simulink model "suivi_points"  (R2021b)
settings: Solver=VariableStepAuto  StartTime=0.0  StopTime=100.0  RelTol=1e-3
values from neighbouring files (symbols this model uses):
  a1mot = -lambdamot    [fichierconfig.m]
  alphainit = 3.14/2    (= 1.57)    [fichierconfig.m]
  b1mot = G*(1-lambdamot)    [fichierconfig.m]
  L = 0.0865    [fichierconfig.m]
  paramIangle = (r1angle+r0angle)/Te    (= 1.25)    [fichierconfig.m]
  paramImoteur = (r1+r0)/Te    (= 2.95980583674)    [fichierconfig.m]
  paramPangle = r0angle    (= 0.1625)    [fichierconfig.m]
  paramPmoteur = r0    (= 0.384774758776)    [fichierconfig.m]
  Pxcible = +0.5    (= 0.5)    [fichierconfig.m]
  Pxinit = 0    [fichierconfig.m]
  Pycible = -0.5    [fichierconfig.m]
  Pyinit = 0    [fichierconfig.m]
  r = 0.030    (= 0.03)    [fichierconfig.m]
  Te = 0.040    (= 0.04)    [fichierconfig.m]
undefined symbols (not defined in the file or in its folder): DiscIntNeverNeededParam
libraries: slpidlib x3, simulink x1
settings Model: Creator=mlouaze  LastModifiedBy=mlouaze

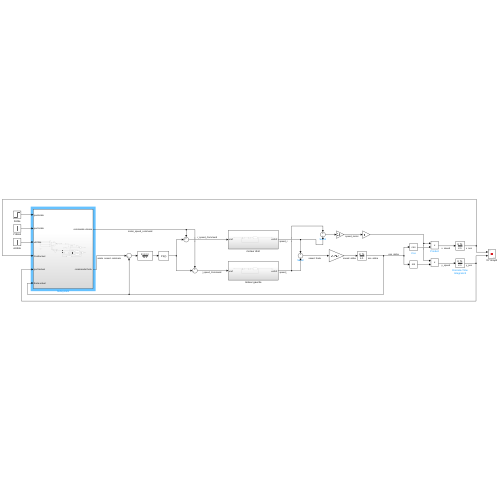
[thumbnail: Simulink's stored preview of the top-level diagram]
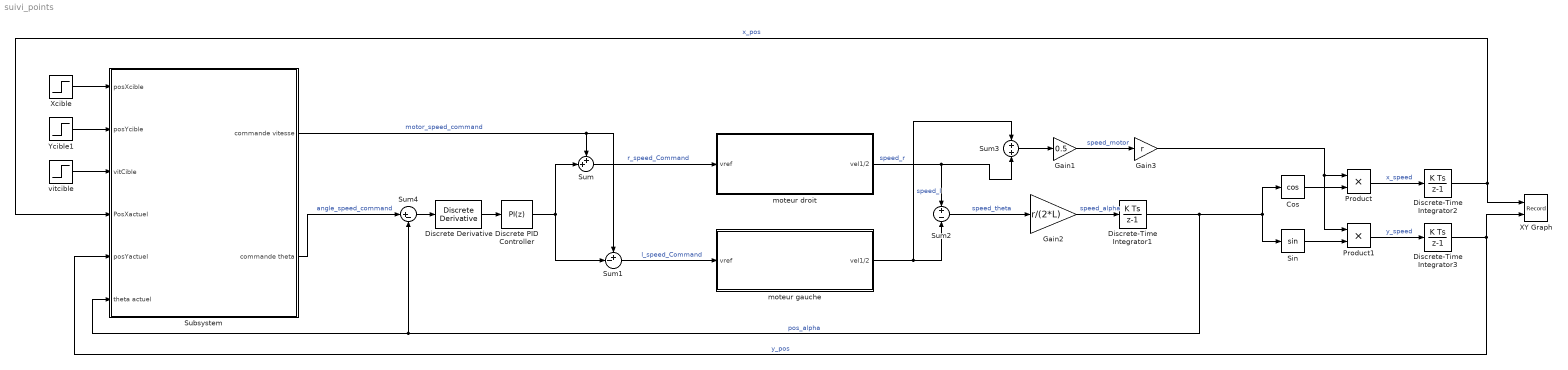
== system suivi_points ==
  Cos : Trigonometry  Operator=cos
  Discrete Derivative : simulink/Discrete/Discrete Derivative  gainval=1.0  ICPrevScaledInput=0.0  OutMin=[]  OutMax=[]  OutDataType=fixdt(1, 16)  OutScaling=2^-10  DoSatur=off
  Discrete PID Controller : slpidlib/PID Controller  Controller=PI  Form=Parallel  TimeDomain=Discrete-time  UseExternalTs=off  SampleTime=-1  IntegratorMethod=Forward Euler  FilterMethod=Forward Euler  ControllerParametersSource=internal  P=paramPangle  I=paramIangle  D=0  UseFilter=on  N=100  TunerSelectOption=Transfer Function Based (PID Tuner App)  InitialConditionSource=internal  InitialConditionForIntegrator=0  InitialConditionForFilter=0  DifferentiatorICPrevScaledInput=0  ExternalReset=none  TrackingMode=off  Kt=1  LimitOutput=off  SatLimitsSource=internal  UpperSaturationLimit=inf  LowerSaturationLimit=-inf  LinearizeAsGain=off  AntiWindupMode=none  Kb=1  POutMin=[]  POutMax=[]  IOutMin=[]  IOutMax=[]  DOutMin=[]  DOutMax=[]  NOutMin=[]  NOutMax=[]  SumOutMin=[]  SumOutMax=[]  SaturationOutMin=[]  SaturationOutMax=[]  PParamMin=[]  PParamMax=[]  IParamMin=[]  IParamMax=[]  DParamMin=[]  DParamMax=[]  NParamMin=[]  NParamMax=[]  KbParamMin=[]  KbParamMax=[]  KtParamMin=[]  KtParamMax=[]  KbOutMin=[]  KbOutMax=[]  KtOutMin=[]  KtOutMax=[]  IntegratorOutMin=[]  IntegratorOutMax=[]  FilterOutMin=[]  FilterOutMax=[]  SumI1OutMin=[]  SumI1OutMax=[]  SumI2OutMin=[]  SumI2OutMax=[]  SumI3OutMin=[]  SumI3OutMax=[]  SumI4OutMin=[]  SumI4OutMax=[]  SumDOutMin=[]  SumDOutMax=[]  DifferentiatorOutMin=[]  DifferentiatorOutMax=[]  FilterDiffOutCoefMin=[]  FilterDiffOutCoefMax=[]  ReciprocalOutMin=[]  ReciprocalOutMax=[]  SumDenOutMin=[]  SumDenOutMax=[]  SumNumOutMin=[]  SumNumOutMax=[]  DivideOutMin=[]  DivideOutMax=[]  UdiffTsProdOutMin=[]  UdiffTsProdOutMax=[]  NTsProdOutMin=[]  NTsProdOutMax=[]  UintegralTsProdOutMin=[]  UintegralTsProdOutMax=[]  UngainTsProdOutMin=[]  UngainTsProdOutMax=[]  IntegratorContinuousStateAttributes=''  IntegratorStateMustResolveToSignalObject=off  IntegratorRTWStateStorageClass=Auto  FilterContinuousStateAttributes=''  FilterStateMustResolveToSignalObject=off  FilterRTWStateStorageClass=Auto  ParallelPVariant=InternalParameters  IdealPVariant=Disabled  IVariant=InternalParameters  DVariant=Disabled  IntegratorVariant=Discrete  SatVariant=Disabled  AWVariant=Passthrough  PCopyVariant=Disabled  TRVariant=Disabled  FdbkBlocksVariant=Forward  IdealPFdbkVariant=Disabled  SatFdbkVariant=Disabled  DerivativeFilterVariant=Disabled  NVariant=Disabled  NCopyVariant=Disabled_SignalSpec  FilterICVariant=Disabled  IntegratorICVariant=InternalICs  ExternalResetVariant=Disabled  TRSumVariant=Passthrough  SumFdbkVariant=Disabled  SumVariant=Sum_PI  TsampFilterVariant=InternalTs  TsampNgainVariant=Passthrough  TsampIntegralVariant=Passthrough  ExternalSaturationOutDataTypeStr=Inherit: Same as second input
  Discrete-Time Integrator1 : DiscreteIntegrator  InitialCondition=alphainit  SampleTime=-1  ICPrevOutput=DiscIntNeverNeededParam  ICPrevScaledInput=DiscIntNeverNeededParam
  Discrete-Time Integrator2 : DiscreteIntegrator  InitialCondition=Pxinit  SampleTime=-1  ICPrevOutput=DiscIntNeverNeededParam  ICPrevScaledInput=DiscIntNeverNeededParam
  Discrete-Time Integrator3 : DiscreteIntegrator  InitialCondition=Pyinit  SampleTime=-1  ICPrevOutput=DiscIntNeverNeededParam  ICPrevScaledInput=DiscIntNeverNeededParam
  Gain1 : Gain  Gain=0.5
  Gain2 : Gain  Gain=r/(2*L)
  Gain3 : Gain  Gain=r
  Product : Product
  Product1 : Product
  Sin : Trigonometry
  Subsystem : Subsystem
  Sum : Sum  Inputs=++|
  Sum1 : Sum  Inputs=+-|
  Sum2 : Sum  Inputs=+|-
  Sum3 : Sum  Inputs=+|+
  Sum4 : Sum  Inputs=|+-
  XY Graph : Record  FileSettingsInternal="{\"entries\":[{\"content\":{\"excelSettings\":{\"content\":{},\"type\":\"Streamout.ExcelSettings\"}},\"type\":\"Streamout.FileSettingStorage\",\"uuid\":\"98866556-d0f7-486d-9cf8-d99074070bc6\"}],\"packageUris\":[\"http://schema.mathworks.com/mf0/streamout_blocks/R2020a\"],\"version\":\"1.0\"}"  Layout=[1 1]  SignalsInternal="{\"entries\":[{\"content\":{\"signals\":[{\"content\":{\"blockPath\":[\"suivi_points/XY Graph\"],\"channel\":[],\"dimensions\":[1],\"domain\":\"suivi_points/XY Graph\",\"lineColor\":\"#a2142f\",\"plots\":[1],\"port\":1,\"sid\":[],\"signalID\":195,\"signalName\":\"x_pos\"},\"type\":\"RecordBlkView.Signal\",\"uuid\":\"87e10cd6-bcd0-46b1-8b3f-b12dfa0b8648\"},{\"content\":{\"blockPath\":[\"suivi_points/XY Graph\"],\"channel\":[],\"dimensions\":[1],\"domain\":\"suivi_points/XY Graph\",\"lineColor\":\"#139fff\",\"plots\":[1],\"port\":2,\"sid\":[],\"signalID\":198,\"signalName\":\"y_pos\"},\"type\":\"RecordBlkView.Signal\",\"uuid\":\"d70f9b69-a242-43ad-b3a3-1026d45bf527\"}]},\"type\":\"RecordBlkView.InputSignals\",\"uuid\":\"c4c30806-3f6a-4c2f-8db3-67a8f3bce1fd\"}],\"packageUris\":[\"http://schema.mathworks.com/mf0/streamout_blocks/R2020a\"],\"version\":\"1.0\"}"  VisualizationBindings="{\"xyplotplugin\":{\"info\":[{\"series\":[{\"bindingParametersList\":[{\"parameter\":\"X-Axis\",\"signalID\":195,\"signalName\":\"x_pos\"},{\"parameter\":\"Y-Axis\",\"signalID\":198,\"signalName\":\"y_pos\"}],\"seriesID\":64413}],\"subplotID\":1}]}}"  CompatibilityTag=XY  st=-1
  Xcible : Step  Time=0  After=Pxcible  SampleTime=Te
  Ycible1 : Step  Time=0  After=Pycible  SampleTime=Te
  moteur droit : Subsystem
  moteur gauche : Subsystem
  vitcible : Step  Time=0  SampleTime=Te
  wires:
  Sum3/1 -> Gain1/1
  Xcible/1 -> Subsystem/1(posXcible)
  Cos/1 -> Product/2
  Ycible1/1 -> Subsystem/2(posYcible)
  Sum2/1 -> Gain2/1  "speed_theta"
  Product/1 -> Discrete-Time Integrator2/1  "x_speed"
  Subsystem/1(commande vitesse) -> Sum1/1, Sum/1  "motor_speed_command"
  Discrete PID Controller/1 -> Sum/2, Sum1/2
  Subsystem/2("commande theta ") -> Sum4/1  "angle_speed_command"
  moteur droit/1(vel1/2) -> Sum3/2, Sum2/1  "speed_r"
  moteur gauche/1(vel1/2) -> Sum2/2, Sum3/1  "speed_l"
  Discrete-Time Integrator1/1 -> Cos/1, Sin/1, Subsystem/6(theta actuel), Sum4/2  "pos_alpha"
  Gain2/1 -> Discrete-Time Integrator1/1  "speed_alpha"
  Discrete-Time Integrator3/1 -> XY Graph/2, Subsystem/5(posYactuel)  "y_pos"
  Sum1/1 -> moteur gauche/1(vref)  "l_speed_Command"
  Sin/1 -> Product1/2
  Sum/1 -> moteur droit/1(vref)  "r_speed_Command"
  Gain3/1 -> Product1/1, Product/1
  Product1/1 -> Discrete-Time Integrator3/1  "y_speed"
  Discrete-Time Integrator2/1 -> XY Graph/1, Subsystem/4(PosXactuel)  "x_pos"
  Gain1/1 -> Gain3/1  "speed_motor"
  vitcible/1 -> Subsystem/3(vitCible)
  Discrete Derivative/1 -> Discrete PID Controller/1
  Sum4/1 -> Discrete Derivative/1

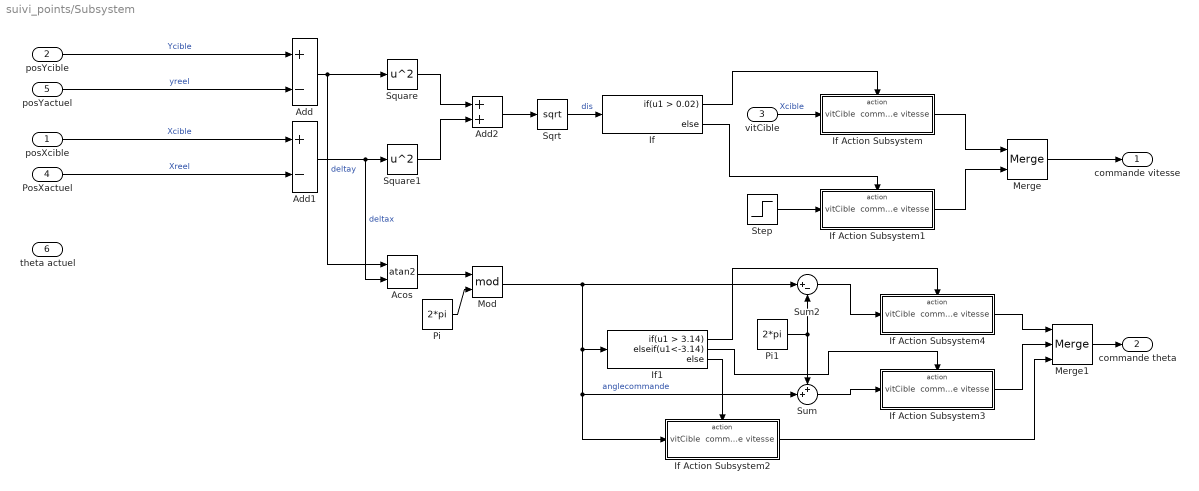
== system suivi_points/Subsystem ==
  posXcible : Inport
  posYcible : Inport  Port=2
  vitCible : Inport  Port=3
  PosXactuel : Inport  Port=4
  posYactuel : Inport  Port=5
  theta actuel : Inport  Port=6
  Acos : Trigonometry  Operator=atan2
  Add : Sum  Inputs=+-
  Add1 : Sum  Inputs=+-
  Add2 : Sum
  If : If  IfExpression=u1 > 0.02
  If Action Subsystem : Subsystem  TreatAsAtomicUnit=on
  If Action Subsystem1 : Subsystem  TreatAsAtomicUnit=on
  If Action Subsystem2 : Subsystem  TreatAsAtomicUnit=on
  If Action Subsystem3 : Subsystem  TreatAsAtomicUnit=on
  If Action Subsystem4 : Subsystem  TreatAsAtomicUnit=on
  If1 : If  IfExpression=u1 > 3.14  ElseIfExpressions=u1<-3.14
  Merge : Merge
  Merge1 : Merge  Inputs=3
  Mod : Math  Operator=mod  SaturateOnIntegerOverflow=on
  Pi : Constant  Value=2*pi  OutDataTypeStr=Inherit: Inherit via back propagation  SampleTime=-1
  Pi1 : Constant  Value=2*pi  OutDataTypeStr=Inherit: Inherit via back propagation
  Sqrt : Sqrt  SaturateOnIntegerOverflow=on
  Square : Math  Operator=square  SaturateOnIntegerOverflow=on
  Square1 : Math  Operator=square  SaturateOnIntegerOverflow=on
  Step : Step  Time=0  After=0  SampleTime=0
  Sum : Sum  Inputs=++|
  Sum2 : Sum  Inputs=|+-
  commande vitesse : Outport
  "commande theta " : Outport  Port=2
  wires:
  posYcible/1 -> Add/1  "Ycible"
  posYactuel/1 -> Add/2  "yreel"
  posXcible/1 -> Add1/1  "Xcible"
  PosXactuel/1 -> Add1/2  "Xreel"
  Add/1 -> Acos/1, Square/1  "deltay"
  Add1/1 -> Square1/1, Acos/2  "deltax"
  Square1/1 -> Add2/2
  Square/1 -> Add2/1
  Add2/1 -> Sqrt/1
  Sqrt/1 -> If/1  "dis"
  Mod/1 -> If Action Subsystem2/1(vitCible), Sum/2, If1/1, Sum2/1  "anglecommande"
  Merge1/1 -> "commande theta "/1
  vitCible/1 -> If Action Subsystem/1(vitCible)  "Xcible"
  If/1 -> If Action Subsystem/Action
  If/2 -> If Action Subsystem1/Action
  Step/1 -> If Action Subsystem1/1(vitCible)
  Merge/1 -> commande vitesse/1
  If Action Subsystem1/1(commande vitesse) -> Merge/2
  Acos/1 -> Mod/1
  Pi/1 -> Mod/2
  If1/3 -> If Action Subsystem2/Action
  If Action Subsystem2/1(commande vitesse) -> Merge1/3
  If1/2 -> If Action Subsystem3/Action
  If Action Subsystem3/1(commande vitesse) -> Merge1/2
  Sum/1 -> If Action Subsystem3/1(vitCible)
  If1/1 -> If Action Subsystem4/Action
  If Action Subsystem4/1(commande vitesse) -> Merge1/1
  Sum2/1 -> If Action Subsystem4/1(vitCible)
  Pi1/1 -> Sum/1, Sum2/2
  If Action Subsystem/1(commande vitesse) -> Merge/1

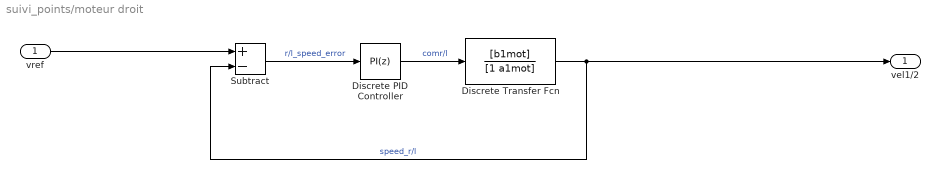
== system suivi_points/moteur droit ==
  vref : Inport
  Discrete Transfer Fcn : DiscreteTransferFcn  Numerator=[b1mot]  Denominator=[1 a1mot]
  Discrete PID Controller : slpidlib/PID Controller  Controller=PI  Form=Parallel  TimeDomain=Discrete-time  UseExternalTs=off  SampleTime=-1  IntegratorMethod=Forward Euler  FilterMethod=Forward Euler  ControllerParametersSource=internal  P=paramPmoteur  I=paramImoteur  D=0  UseFilter=on  N=100  TunerSelectOption=Transfer Function Based (PID Tuner App)  InitialConditionSource=internal  InitialConditionForIntegrator=0  InitialConditionForFilter=0  DifferentiatorICPrevScaledInput=0  ExternalReset=none  TrackingMode=off  Kt=1  LimitOutput=off  SatLimitsSource=internal  UpperSaturationLimit=inf  LowerSaturationLimit=-inf  LinearizeAsGain=off  AntiWindupMode=none  Kb=1  POutMin=[]  POutMax=[]  IOutMin=[]  IOutMax=[]  DOutMin=[]  DOutMax=[]  NOutMin=[]  NOutMax=[]  SumOutMin=[]  SumOutMax=[]  SaturationOutMin=[]  SaturationOutMax=[]  PParamMin=[]  PParamMax=[]  IParamMin=[]  IParamMax=[]  DParamMin=[]  DParamMax=[]  NParamMin=[]  NParamMax=[]  KbParamMin=[]  KbParamMax=[]  KtParamMin=[]  KtParamMax=[]  KbOutMin=[]  KbOutMax=[]  KtOutMin=[]  KtOutMax=[]  IntegratorOutMin=[]  IntegratorOutMax=[]  FilterOutMin=[]  FilterOutMax=[]  SumI1OutMin=[]  SumI1OutMax=[]  SumI2OutMin=[]  SumI2OutMax=[]  SumI3OutMin=[]  SumI3OutMax=[]  SumI4OutMin=[]  SumI4OutMax=[]  SumDOutMin=[]  SumDOutMax=[]  DifferentiatorOutMin=[]  DifferentiatorOutMax=[]  FilterDiffOutCoefMin=[]  FilterDiffOutCoefMax=[]  ReciprocalOutMin=[]  ReciprocalOutMax=[]  SumDenOutMin=[]  SumDenOutMax=[]  SumNumOutMin=[]  SumNumOutMax=[]  DivideOutMin=[]  DivideOutMax=[]  UdiffTsProdOutMin=[]  UdiffTsProdOutMax=[]  NTsProdOutMin=[]  NTsProdOutMax=[]  UintegralTsProdOutMin=[]  UintegralTsProdOutMax=[]  UngainTsProdOutMin=[]  UngainTsProdOutMax=[]  IntegratorContinuousStateAttributes=''  IntegratorStateMustResolveToSignalObject=off  IntegratorRTWStateStorageClass=Auto  FilterContinuousStateAttributes=''  FilterStateMustResolveToSignalObject=off  FilterRTWStateStorageClass=Auto  ParallelPVariant=InternalParameters  IdealPVariant=Disabled  IVariant=InternalParameters  DVariant=Disabled  IntegratorVariant=Discrete  SatVariant=Disabled  AWVariant=Passthrough  PCopyVariant=Disabled  TRVariant=Disabled  FdbkBlocksVariant=Forward  IdealPFdbkVariant=Disabled  SatFdbkVariant=Disabled  DerivativeFilterVariant=Disabled  NVariant=Disabled  NCopyVariant=Disabled_SignalSpec  FilterICVariant=Disabled  IntegratorICVariant=InternalICs  ExternalResetVariant=Disabled  TRSumVariant=Passthrough  SumFdbkVariant=Disabled  SumVariant=Sum_PI  TsampFilterVariant=InternalTs  TsampNgainVariant=Passthrough  TsampIntegralVariant=Passthrough  ExternalSaturationOutDataTypeStr=Inherit: Same as second input
  Subtract : Sum  Inputs=+-
  vel1/2 : Outport
  wires:
  vref/1 -> Subtract/1
  Discrete Transfer Fcn/1 -> Subtract/2, vel1/2/1  "speed_r/l"
  Discrete PID Controller/1 -> Discrete Transfer Fcn/1  "comr/l"
  Subtract/1 -> Discrete PID Controller/1  "r/l_speed_error"

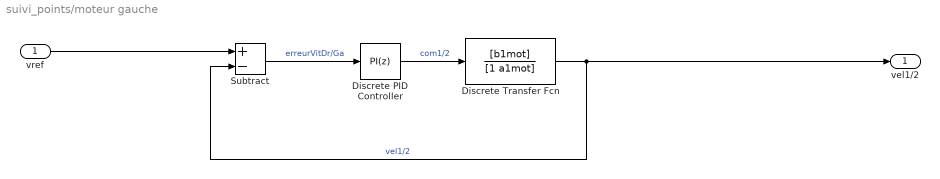
== system suivi_points/moteur gauche ==
  vref : Inport
  Discrete Transfer Fcn : DiscreteTransferFcn  Numerator=[b1mot]  Denominator=[1 a1mot]
  Discrete PID Controller : slpidlib/PID Controller  Controller=PI  Form=Parallel  TimeDomain=Discrete-time  UseExternalTs=off  SampleTime=-1  IntegratorMethod=Forward Euler  FilterMethod=Forward Euler  ControllerParametersSource=internal  P=paramPmoteur  I=paramImoteur  D=0  UseFilter=on  N=100  TunerSelectOption=Transfer Function Based (PID Tuner App)  InitialConditionSource=internal  InitialConditionForIntegrator=0  InitialConditionForFilter=0  DifferentiatorICPrevScaledInput=0  ExternalReset=none  TrackingMode=off  Kt=1  LimitOutput=off  SatLimitsSource=internal  UpperSaturationLimit=inf  LowerSaturationLimit=-inf  LinearizeAsGain=off  AntiWindupMode=none  Kb=1  POutMin=[]  POutMax=[]  IOutMin=[]  IOutMax=[]  DOutMin=[]  DOutMax=[]  NOutMin=[]  NOutMax=[]  SumOutMin=[]  SumOutMax=[]  SaturationOutMin=[]  SaturationOutMax=[]  PParamMin=[]  PParamMax=[]  IParamMin=[]  IParamMax=[]  DParamMin=[]  DParamMax=[]  NParamMin=[]  NParamMax=[]  KbParamMin=[]  KbParamMax=[]  KtParamMin=[]  KtParamMax=[]  KbOutMin=[]  KbOutMax=[]  KtOutMin=[]  KtOutMax=[]  IntegratorOutMin=[]  IntegratorOutMax=[]  FilterOutMin=[]  FilterOutMax=[]  SumI1OutMin=[]  SumI1OutMax=[]  SumI2OutMin=[]  SumI2OutMax=[]  SumI3OutMin=[]  SumI3OutMax=[]  SumI4OutMin=[]  SumI4OutMax=[]  SumDOutMin=[]  SumDOutMax=[]  DifferentiatorOutMin=[]  DifferentiatorOutMax=[]  FilterDiffOutCoefMin=[]  FilterDiffOutCoefMax=[]  ReciprocalOutMin=[]  ReciprocalOutMax=[]  SumDenOutMin=[]  SumDenOutMax=[]  SumNumOutMin=[]  SumNumOutMax=[]  DivideOutMin=[]  DivideOutMax=[]  UdiffTsProdOutMin=[]  UdiffTsProdOutMax=[]  NTsProdOutMin=[]  NTsProdOutMax=[]  UintegralTsProdOutMin=[]  UintegralTsProdOutMax=[]  UngainTsProdOutMin=[]  UngainTsProdOutMax=[]  IntegratorContinuousStateAttributes=''  IntegratorStateMustResolveToSignalObject=off  IntegratorRTWStateStorageClass=Auto  FilterContinuousStateAttributes=''  FilterStateMustResolveToSignalObject=off  FilterRTWStateStorageClass=Auto  ParallelPVariant=InternalParameters  IdealPVariant=Disabled  IVariant=InternalParameters  DVariant=Disabled  IntegratorVariant=Discrete  SatVariant=Disabled  AWVariant=Passthrough  PCopyVariant=Disabled  TRVariant=Disabled  FdbkBlocksVariant=Forward  IdealPFdbkVariant=Disabled  SatFdbkVariant=Disabled  DerivativeFilterVariant=Disabled  NVariant=Disabled  NCopyVariant=Disabled_SignalSpec  FilterICVariant=Disabled  IntegratorICVariant=InternalICs  ExternalResetVariant=Disabled  TRSumVariant=Passthrough  SumFdbkVariant=Disabled  SumVariant=Sum_PI  TsampFilterVariant=InternalTs  TsampNgainVariant=Passthrough  TsampIntegralVariant=Passthrough  ExternalSaturationOutDataTypeStr=Inherit: Same as second input
  Subtract : Sum  Inputs=+-
  vel1/2 : Outport
  wires:
  vref/1 -> Subtract/1
  Discrete Transfer Fcn/1 -> Subtract/2, vel1/2/1  "vel1/2"
  Discrete PID Controller/1 -> Discrete Transfer Fcn/1  "com1/2"
  Subtract/1 -> Discrete PID Controller/1  "erreurVitDr/Ga"

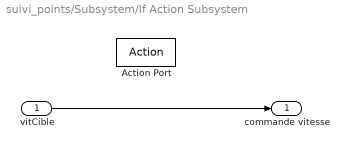
== system suivi_points/Subsystem/If Action Subsystem ==
  vitCible : Inport
  Action Port : ActionPort  ActionPortLabel=if(u1 > 0.02)
  commande vitesse : Outport
  wires:
  vitCible/1 -> commande vitesse/1

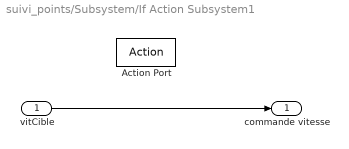
== system suivi_points/Subsystem/If Action Subsystem1 ==
  vitCible : Inport
  Action Port : ActionPort  ActionPortLabel=else
  commande vitesse : Outport
  wires:
  vitCible/1 -> commande vitesse/1

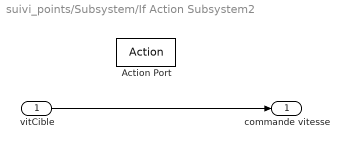
== system suivi_points/Subsystem/If Action Subsystem2 ==
  vitCible : Inport
  Action Port : ActionPort  ActionPortLabel=else
  commande vitesse : Outport
  wires:
  vitCible/1 -> commande vitesse/1

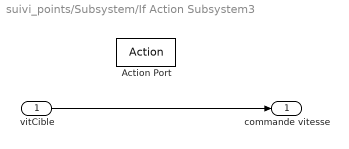
== system suivi_points/Subsystem/If Action Subsystem3 ==
  vitCible : Inport
  Action Port : ActionPort  ActionPortLabel=elseif(u1<-3.14)
  commande vitesse : Outport
  wires:
  vitCible/1 -> commande vitesse/1

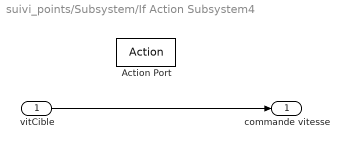
== system suivi_points/Subsystem/If Action Subsystem4 ==
  vitCible : Inport
  Action Port : ActionPort  ActionPortLabel=if(u1 > 3.14)
  commande vitesse : Outport
  wires:
  vitCible/1 -> commande vitesse/1
